simulink model "Output_Feedback"  (R2022b)
settings: Solver=FixedStepAuto  StartTime=0.0  StopTime=430  FixedStep=step_size  RelTol=1e-3
undefined symbols (not defined in the file): b, unicycle
libraries: simulink_extras x1
settings Model: Creator=Musta  LastModifiedBy=Musta

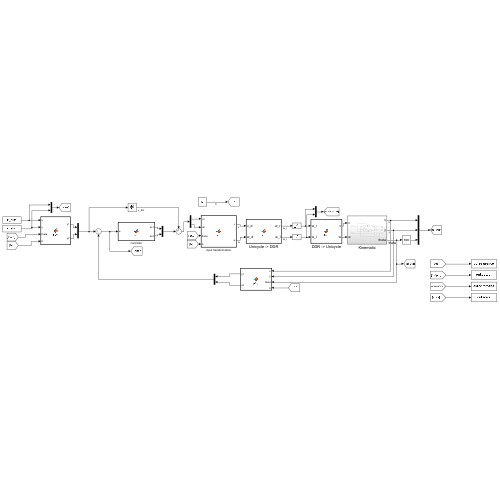
[thumbnail: Simulink's stored preview of the top-level diagram]
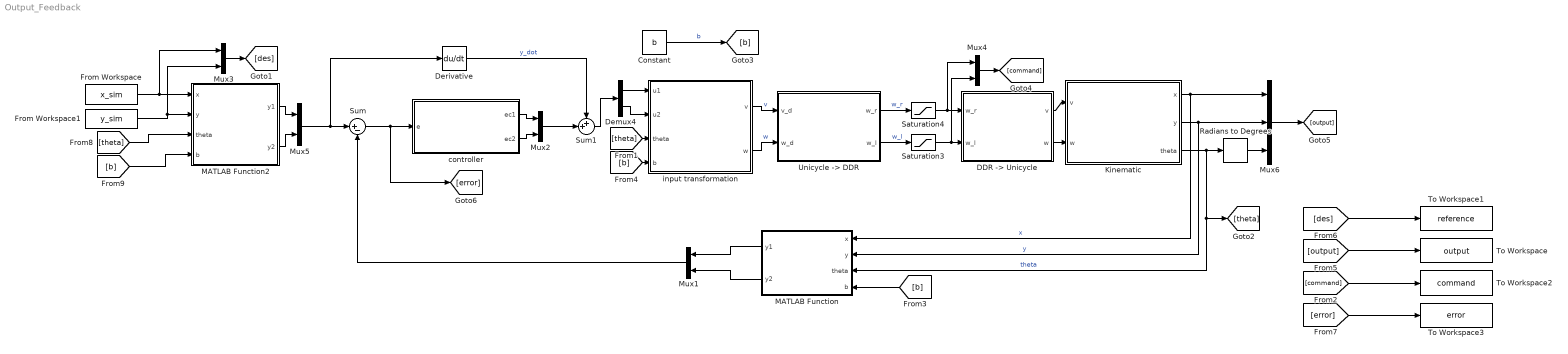
== system Output_Feedback ==
  " DDR -> Unicycle " : MATLAB Function  TreatAsAtomicUnit=on
  Constant : Constant  Value=b
  Demux4 : Demux  Outputs=2
  Derivative : Derivative
  From Workspace : FromWorkspace  VariableName=x_sim
  From Workspace1 : FromWorkspace  VariableName=y_sim
  Kinematic : Subsystem
  MATLAB Function : MATLAB Function  TreatAsAtomicUnit=on
  MATLAB Function2 : MATLAB Function  TreatAsAtomicUnit=on
  Mux{1..5} (5 alike) : Mux  Inputs=2
  Mux6 : Mux  Inputs=3
  Radians to Degrees : simulink_extras/Transformations/Radians to Degrees
  Saturation3 : Saturate  UpperLimit=unicycle.omegaWheelMax  LowerLimit=unicycle.omegaWheelMin
  Saturation4 : Saturate  UpperLimit=unicycle.omegaWheelMax  LowerLimit=unicycle.omegaWheelMin
  Sum : Sum  Inputs=|+-
  Sum1 : Sum  Inputs=++|
  To Workspace : ToWorkspace  VariableName=output  SaveFormat=Structure With Time  SampleTime=-1
  To Workspace1 : ToWorkspace  VariableName=reference  SaveFormat=Structure With Time  SampleTime=-1
  To Workspace2 : ToWorkspace  VariableName=command  SaveFormat=Structure With Time  SampleTime=-1
  To Workspace3 : ToWorkspace  VariableName=error  SaveFormat=Structure With Time  SampleTime=-1
  "Unicycle -> DDR" : MATLAB Function  TreatAsAtomicUnit=on
  controller : MATLAB Function  TreatAsAtomicUnit=on
  input transformation : MATLAB Function  TreatAsAtomicUnit=on
  wires:
  From Workspace/1 -> Mux3/1, MATLAB Function2/1(x)
  Mux3/1 -> [des]
  [theta] -> MATLAB Function2/3(theta)
  Mux1/1 -> Sum/2
  From Workspace1/1 -> Mux3/2, MATLAB Function2/2(y)
  MATLAB Function2/2(y2) -> Mux5/2
  [b] -> MATLAB Function/4(b)
  MATLAB Function/2(y2) -> Mux1/2
  MATLAB Function2/1(y1) -> Mux5/1
  [b] -> MATLAB Function2/4(b)
  Derivative/1 -> Sum1/1  "y_dot"
  Mux5/1 -> Derivative/1, Sum/1
  Demux4/1 -> input transformation/1(u1)
  [theta] -> input transformation/3(theta)
  Demux4/2 -> input transformation/2(u2)
  controller/1(ec1) -> Mux2/1
  Mux2/1 -> Sum1/2
  input transformation/1(v) -> "Unicycle -> DDR"/1(v_d)  "v"
  Constant/1 -> [b]  "b"
  Sum1/1 -> Demux4/1
  controller/2(ec2) -> Mux2/2
  MATLAB Function/1(y1) -> Mux1/1
  [b] -> input transformation/4(b)
  input transformation/2(w) -> "Unicycle -> DDR"/2(w_d)  "w"
  Kinematic/2(y) -> Mux6/2, MATLAB Function/2(y)  "y"
  Saturation3/1 -> Mux4/2, " DDR -> Unicycle "/2(w_l)
  "Unicycle -> DDR"/2(w_l) -> Saturation3/1  "w_l"
  " DDR -> Unicycle "/2(w) -> Kinematic/2(w)
  Mux4/1 -> [command]
  Kinematic/3(theta) -> [theta], MATLAB Function/3(theta), Radians to Degrees/1  "theta"
  Saturation4/1 -> " DDR -> Unicycle "/1(w_r), Mux4/1
  "Unicycle -> DDR"/1(w_r) -> Saturation4/1  "w_r"
  [command] -> To Workspace2/1
  Mux6/1 -> [output]
  Kinematic/1(x) -> Mux6/1, MATLAB Function/1(x)  "x"
  [des] -> To Workspace1/1
  Radians to Degrees/1 -> Mux6/3
  " DDR -> Unicycle "/1(v) -> Kinematic/1(v)
  [output] -> To Workspace/1
  Sum/1 -> [error], controller/1(e)
  [error] -> To Workspace3/1

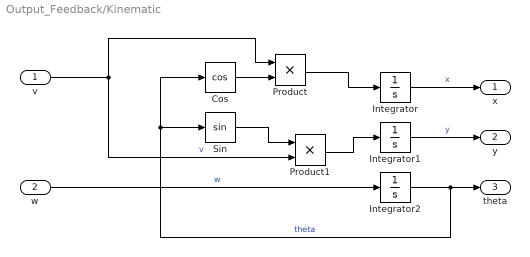
== system Output_Feedback/Kinematic ==
  v : Inport
  w : Inport  Port=2
  Cos : Trigonometry  Operator=cos
  Integrator : Integrator  InitialCondition=unicycle.ic.x
  Integrator1 : Integrator  InitialCondition=unicycle.ic.y
  Integrator2 : Integrator  InitialCondition=unicycle.ic.theta
  Product : Product
  Product1 : Product
  Sin : Trigonometry
  x : Outport
  y : Outport  Port=2
  theta : Outport  Port=3
  wires:
  w/1 -> Integrator2/1  "w"
  Product/1 -> Integrator/1
  v/1 -> Product/1, Product1/2  "v"
  Cos/1 -> Product/2
  Integrator1/1 -> y/1  "y"
  Integrator/1 -> x/1  "x"
  Integrator2/1 -> Cos/1, Sin/1, theta/1  "theta"
  Product1/1 -> Integrator1/1
  Sin/1 -> Product1/1

== matlab function Output_Feedback/MATLAB Function2 ==
  data: x input; y1 output; y input; y2 output; theta input; b input
function [y1,y2] = p2y(x,y,theta,b)

y1 = x + b*cos(theta);
y2 = y + b*sin(theta);

== matlab function Output_Feedback/input transformation ==
  data: u1 input; u2 input; theta input; v output; b input; w output
function [v,w] = fcn(u1, u2, theta, b)

    R = [cos(theta),      sin(theta);
         -sin(theta)/b, cos(theta)/b];
    
    v = cos(theta)*u1 + sin(theta)*u2;
    w = (-sin(theta)/b)*u1 + (cos(theta)/b)*u2;

end

== matlab function Output_Feedback/MATLAB Function ==
  data: x input; y1 output; y input; theta input; b input; y2 output
function [y1,y2] = p2y(x,y,theta,b)

    y1 = x + b*cos(theta);
    y2 = y + b*sin(theta);
    
end

== matlab function Output_Feedback/controller ==
  data: e input; ec1 output; ec2 output
function [ec1, ec2] = fcn(e)

    %#codegen
    coder.extrinsic('evalin')
    k1 = 0;                  % Needed in order to set variable class correctly
    k2 = 0;                  % Needed in order to set variable class correctly
    k1 = evalin('base','k1'); % Read value from workspace
    k2 = evalin('base','k2'); % Read value from workspace
    
    ec1 = k1*(e(1));
    ec2 = k2*(e(2));
    
end

== matlab function Output_Feedback/ DDR -> Unicycle  ==
  data: w_r input; v output; w_l input; w output
function [v, w] = fcn(w_r, w_l)

    %#codegen
    coder.extrinsic('evalin')
    d = 0;                  % Needed in order to set variable class correctly
    r = 0;                  % Needed in order to set variable class correctly
    d = evalin('base','unicycle.d'); % Read value from workspace
    r = evalin('base','unicycle.r'); % Read value from workspace

    v = r*(w_r + w_l)/2; % rad/s
    w = r*(w_r - w_l)/d; % rad/s

end

== matlab function Output_Feedback/Unicycle -> DDR ==
  data: v_d input; w_r output; w_d input; w_l output
function [w_r, w_l] = fcn(v_d, w_d)

    %#codegen
    coder.extrinsic('evalin')
    d = 0;                  % Needed in order to set variable class correctly
    r = 0;                  % Needed in order to set variable class correctly
    d = evalin('base','unicycle.d'); % Read value from workspace
    r = evalin('base','unicycle.r'); % Read value from workspace

    w_r = ((2 * v_d) + (w_d * d)) / (2 * r);
    w_l = ((2 * v_d) - (w_d * d)) / (2 * r);

end
